simulink model "forceField_sim"  (R2023a)
settings: Solver=FixedStepAuto  StartTime=0.0  StopTime=inf  FixedStep=time_step  RelTol=1e-3
InitFcn:
  | reaching_init
values from neighbouring files (symbols this model uses):
  coord_home = [0,0]    [reaching_init.m]
  coord_targets = zeros(n_target,2)    [reaching_init.m]
  th = 0.005    [reaching_init.m]
libraries: simulink x1, vrlib x1
settings Model: Creator=davide  LastModifiedBy=davide

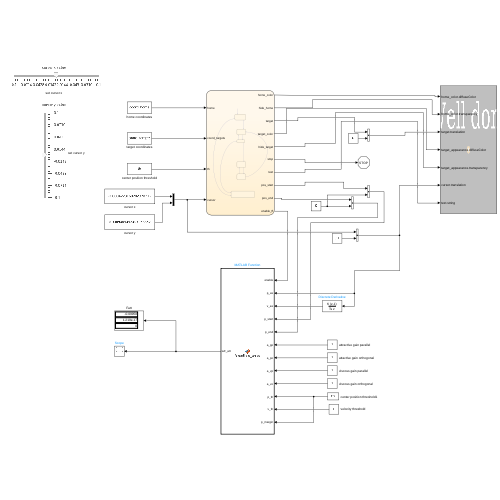
[thumbnail: Simulink's stored preview of the top-level diagram]
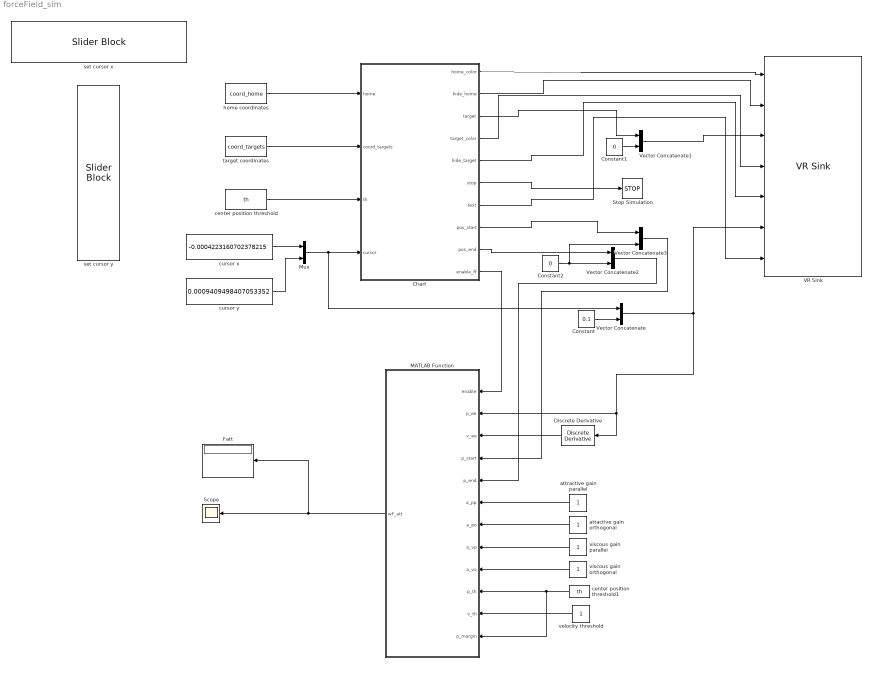
== system forceField_sim ==
  Chart : Stateflow chart  TreatAsAtomicUnit=on
  Constant : Constant  Value=0.1
  Constant1 : Constant  Value=0
  Constant2 : Constant  Value=0
  Discrete Derivative : simulink/Discrete/Discrete Derivative  gainval=1.0  ICPrevScaledInput=0.0  OutMin=[]  OutMax=[]  OutDataType=fixdt(1, 16)  OutScaling=2^-10  DoSatur=off
  Fatt : Display
  MATLAB Function : MATLAB Function  TreatAsAtomicUnit=on
  Mux : Mux  Inputs=2
  Scope : Scope
  Stop Simulation : Stop
  VR Sink : vrlib/VR Sink  InstantiateOnLoad=on  SampleTime=0.1  ViewEnable=on  RemoteChange=off  RemoteView=off  FieldsWritten=home_color.diffuseColor.3.1.1.double#home_color.transparency.1.1.1.double#target.translation.3.1.1.double#target_appearance.diffuseColor.3.1.1.double#target_appearance.transparency.1.1.1.double#cursor.translation.3.1.1.double#text.string.1.-1.1.char  WorldFileName=a3_world.wrl  AutoView=off  VideoDimensions=[]  AllowVariableSize=off  FigureProperties="{'Position', 'Name', 'Viewpoint', 'CameraBound', 'CameraDirection', 'CameraPosition', 'CameraUpVector', 'ZoomFactor', 'Antialiasing', 'Headlight', 'Lighting', 'NavPanel', 'Sound', 'StatusBar', 'Stereo3D', 'Stereo3DCameraOffset', 'Stereo3DHIT', 'ToolBar', 'Textures', 'Transparency', 'Triad', 'Wireframe', 'NavZones', 'NavMode', 'NavSpeed', 'CaptureFileFormat', 'CaptureFileName', 'Record2DCompressMethod', 'Record2DCompressQuality', 'Record2D', 'Record2DFileName', 'Record2DFPS'; [7.1000000000000000e+01   1.1800000000000000e+02   5.7600000000000000e+02   3.5000000000000000e+02], '', 'default', 'on', [0.0000000000000000e+00   0.0000000000000000e+00  -1.0000000000000000e+00], [0.0000000000000000e+00   0.0000000000000000e+00   0.0000000000000000e+00], [0.0000000000000000e+00   1.0000000000000000e+00   0.0000000000000000e+00], [1.0000000000000000e+00], 'on', 'on', 'on', 'halfbar', 'on', 'on', 'off', [1.0000000149011612e-01], [0.0000000000000000e+00], 'on', 'on', 'on', 'none', 'off', 'off', 'fly', 'normal', 'tif', '%f_anim_%n.tif', 'auto', [7.5000000000000000e+01], 'off', '%f_anim_%n.avi', 'auto'}"
  Vector Concatenate{,1..3} (4 alike) : Concatenate
  attactive gain orthogonal : Constant
  attractive gain parallel : Constant
  center position threshold : Constant  Value=th
  center position threshold1 : Constant  Value=th
  cursor x : Constant  Value=-0.0004223160702378215
  cursor y : Constant  Value=0.0009409498407053352
  home coordinates : Constant  Value=coord_home
  set cursor x : SliderBlock  ScaleMin=-0.1  ScaleMax=0.1
  set cursor y : SliderBlock  ScaleMin=-0.1  ScaleMax=0.1
  target coordinates : Constant  Value=coord_targets
  velocity threshold : Constant
  viscous gain orthogonal : Constant
  viscous gain parallel : Constant
  wires:
  target coordinates/1 -> Chart/2(coord_targets)
  center position threshold/1 -> Chart/3(th)
  home coordinates/1 -> Chart/1(home)
  cursor x/1 -> Mux/1
  cursor y/1 -> Mux/2
  Mux/1 -> Vector Concatenate/1, Chart/4(cursor)
  Constant/1 -> Vector Concatenate/2
  Constant1/1 -> Vector Concatenate1/2
  Chart/3(target) -> Vector Concatenate1/1
  Chart/6(stop) -> Stop Simulation/1
  Chart/2(hide_home) -> VR Sink/2
  Vector Concatenate1/1 -> VR Sink/3
  Chart/4(target_color) -> VR Sink/4
  Chart/5(hide_target) -> VR Sink/5
  Chart/7(text) -> VR Sink/7
  Chart/1(home_color) -> VR Sink/1
  Discrete Derivative/1 -> MATLAB Function/3(v_ee)
  attractive gain parallel/1 -> MATLAB Function/6(a_pp)
  attactive gain orthogonal/1 -> MATLAB Function/7(a_po)
  viscous gain parallel/1 -> MATLAB Function/8(a_vp)
  viscous gain orthogonal/1 -> MATLAB Function/9(a_vo)
  velocity threshold/1 -> MATLAB Function/11(v_th)
  MATLAB Function/1(wF_att) -> Scope/1, Fatt/1
  Vector Concatenate/1 -> Discrete Derivative/1, MATLAB Function/2(p_ee), VR Sink/6
  Chart/8(pos_start) -> Vector Concatenate3/1
  Chart/9(pos_end) -> Vector Concatenate2/1
  Constant2/1 -> Vector Concatenate3/2, Vector Concatenate2/2
  Vector Concatenate2/1 -> MATLAB Function/5(p_end)
  Vector Concatenate3/1 -> MATLAB Function/4(p_start)
  center position threshold1/1 -> MATLAB Function/12(p_margin), MATLAB Function/10(p_th)
  Chart/10(enable_ff) -> MATLAB Function/1(enable)

== matlab function forceField_sim/MATLAB Function ==
  data: enable input; p_ee input; wF_att output; v_ee input; p_start input; p_end input; a_pp input; a_po input; a_vp input; a_vo input; p_th input; v_th input; p_margin input
%%
% Generates a force field to attract the manipulator end-effector to a goal
% position proportional to the distance and an anisotorpic viscousity,
% stronger on the orthogonal direction to the distance.
% If the end-effector position is outside a threshold with respect to the
% ideal linear trajectory, a resistive force  proportional with respect to 
% the distance from the ideal trajectory is applied to bring back the
% end-effector closer to the ideal trajectory.
% Home position is considered the origin at (0,0)
%
% NOTE:
% position in meter [m]
% velocity in meter/second [m/s]
%
% Notation:
%   p_ee = end-effector position (vector, 3x1)
%   v_ee = end-effector velocity (vector, 3x1)
%   p_g = goal position (vector, 3x1)
%   v_g = goal velocity (vector, 3x1)
%   a_pp = position error gain parallel (scalar)
%   a_po = position error gain orthogonal (scalar)
%   a_vp = viscosity gain parallel (scalar)
%   a_vo = viscosity gain orthogonal (scalar)
%   
%   p_margin = margin before apply direction compensation
%
% The attractive force is considered only on the plane, thus the following
% projector is considered:
%        
%   Rxy = [1 0 0;
%          0 1 0;
%          0 0 0]
%
% The coordinates will be projected in the plane using such an operator.
% Define distance frame with x-axis along the direction of the distance
% vector between the goal and home, y-axis orthogonal right-handed to it.
%
%   cos(theta) = p_g(1) / norm(p_g)
%   sin(theta) = p_g(2) / norm(p_g)
%
% Rotation matrix to move from world frame to distance frame:
%
%   dRw = [ cos(theta) sin(theta) 0
%          -sin(theta) cos(theta) 0
%                0          0     1]
%
% From now on it is considered to work in distance frame
% The attractive potential is defined as follows:
%
%   U_att = (1/2)*(p_g-p_ee)'*A_p*(p_g-p_ee) + (1/2)*(v_g-v_ee)'*A_v*(v_g-v_ee)
%
% so that the defined Uatt has a minimum at the goal position at zero velocity.
% The attractive force will be the opposite of the attractive potential
% gradient with respect to pee and vee, thus
%
%   F_att = - ∇p_ee(U_att) - ∇v_ee(U_att) = a_p(p_g - p_ee) + a_v(v_g - v_ee)
%
% By hypothesis the goal velocity v_g is null => v_g = 0.
% The resulting actractive force results as follows:
%
%   F_att = (a_p*(p_g-p_ee) - a_v*v_ee)
%
% Thresholds (p_th, v_th) are also considered, after which both
% the position and the velocity errors are considered small enough and the
% target reached.
% The found force needs to be converted into the world frame
%
%   wF_att = dRw'*F_att
%

function wF_att = forceField_aniso(enable, p_ee, v_ee, p_start, p_end, a_pp, a_po, a_vp, a_vo, p_th, v_th, p_margin)
    
    if enable

        % check if input vectors are rows. In case convert them to column
        if isrow(p_ee)
            p_ee = p_ee';
        end
    
        if isrow(v_ee)
            v_ee = v_ee';
        end
    
        if isrow(p_start)
            p_start = p_start';
        end
    
        if isrow(p_end)
            p_end = p_end';
        end
    
    
        % planar projector
        Rxy = [1 0 0;
               0 1 0;
               0 0 0];
    
        % project goal and end-effector coordinates on the plane
        p_end = Rxy*p_end;
        p_ee = Rxy*p_ee;
        v_ee = Rxy*v_ee;
    
        % planar rotation angle between world and distance frame:
        cos_theta = (p_end(1) - p_start(1)) / norm(p_end - p_start);
        sin_theta = (p_end(2) - p_start(2)) / norm(p_end - p_start);
    
        % rotation frame from world to distance frame
        dRw = [ cos_theta sin_theta 0;
               -sin_theta cos_theta 0;
                    0         0     1];
    
        % move from world to distance frame
        dp_end = dRw * p_end;
        dp_ee = dRw * p_ee;
        dv_ee = dRw * v_ee;
    
        % attractive force
        wF_att = zeros(3,1);
    
        % position error matrix gain
        A_p = zeros(3);
        A_p(1,1) = a_pp;
        % check if distance from ideal trajectory is greater than the margin
        if (abs(dp_ee(2)) > p_margin)
            A_p(2,2) = a_po;
        end
    
        % viscous matrix gain
        A_v = zeros(3);
        A_v(1,1) = a_vp;
        A_v(2,2) = a_vo;
    
        if (norm(Rxy*(dp_end - dp_ee)) > p_th) || (norm(Rxy*dv_ee) > v_th)
            % errors greater than thresholds
            wF_att = dRw' * (A_p*(dp_end - dp_ee) - A_v*(dv_ee));
        end
    
    else % force field disabled
        wF_att = [0,0,0]';
    end

== stateflow chart forceField_sim/Chart ==
  state start
  state goToHome
  state home
  state goToTarget
  state target
  state end
    text = string("Well done!");
    enable_ff = false;
    stop = true;
  (default) -> start : {targets = coord_targets;
      |   stop = false;
      |   enable_ff = false;
      |   text = "";}
  start -> end [order 1] : [size(targets,1)==0]
  start -> goToHome [order 2] : {hide_home = false;
      | hide_target = true;
      | home_color = [1,0.6,0];
      | target = home;}
  target -> goToHome [order 2] : after(1,sec)
      | {
      |   hide_target = true;
      |   hide_home = false;
      |   home_color = [1,0.6,0];
      |   pos_start = target;
      |   pos_end = home;
      | }
  home -> goToHome [order 1] : [norm(cursor-home) >= th]
      | {home_color = [1,0.6,0];}
  goToHome -> home : [norm(cursor-home) < th]
      | {home_color = [0,0.8,0];}
  home -> end [order 3] : [size(targets,1) == 0]
  home -> goToTarget [order 2] : after(2,sec)
      | [size(targets,1)>0]
      | {
      |   target = targets(1,1:2)';
      |   targets(1,:) = [];
      |   target_color = [1,0,0];
      |   hide_home = true;
      |   hide_target = false;
      |   pos_start = home;
      |   pos_end = target;
      |   enable_ff = true;
      | }
  target -> goToTarget [order 1] : [norm(cursor-target) >= th]
      | {target_color=[1,0,0];}
  goToTarget -> target : [norm(cursor-target) < th]
      | {
      |   target_color=[0,1,0];
      | }
  data: home_color output; home input; targets local double size=[8,2]; coord_targets input; th input double; cursor input; hide_home output; target output double size=[2,1]; target_color output; hide_target output; stop output; text output string; pos_start output; pos_end output; enable_ff output
